simulink model "AHRS_voter_Harness1"  (R2018b)
settings: Solver=FixedStepDiscrete  StartTime=0.0  StopTime=10.0  FixedStep=0.01  RelTol=1e-3  EnableMultiTasking=on
Description:
  | Testing of a single valid AHRS.
settings Model: Creator=bpotter  LastModifiedBy=bpotter
settings DataIOCC: LimitDataPoints=on  SaveOutput=off  DSMLogging=off  InspectSignalLogs=on  SaveTime=off
settings OptimizationCC: BlockReduction=off  DefaultParameterBehavior=Inlined  InitFltsAndDblsToZero=on  EfficientFloat2IntCast=on  EfficientMapNaN2IntZero=off  LifeSpan=inf  MaxStackSize=inf
settings DebuggingCC: SignalInfNanChecking=error  SignalRangeChecking=error  ReadBeforeWriteMsg=EnableAllAsError  WriteAfterWriteMsg=EnableAllAsError  WriteAfterReadMsg=EnableAllAsError  AlgebraicLoopMsg=error  ArtificialAlgebraicLoopMsg=error  SaveWithDisabledLinksMsg=error  SaveWithParameterizedLinksMsg=error  BlockPriorityViolationMsg=error  SolverPrmCheckMsg=error  InheritedTsInSrcMsg=error  SigSpecEnsureSampleTimeMsg=error  CheckMatrixSingularityMsg=error  IntegerOverflowMsg=error  ParameterUnderflowMsg=error  ParameterPrecisionLossMsg=error  ParameterTunabilityLossMsg=error  UnderSpecifiedDataTypeMsg=error  UnnecessaryDatatypeConvMsg=warning  VectorMatrixConversionMsg=error  SignalLabelMismatchMsg=error  UnconnectedInputMsg=error  UnconnectedOutputMsg=error  UnconnectedLineMsg=error  SFcnCompatibilityMsg=error  BusObjectLabelMismatch=error  RootOutportRequireBusObject=error  AssertControl=DisableAll  AllowSymbolicDim=off  ModelReferenceIOMsg=error  ModelReferenceIOMismatchMessage=error  UnknownTsInhSupMsg=error  ModelReferenceDataLoggingMessage=error  StateNameClashWarn=warning  StrictBusMsg=ErrorOnBusTreatedAsVector  NonBusSignalsTreatedAsBus=error  SFInvalidInputDataAccessInChartInitDiag=error  SFTransitionOutsideNaturalParentDiag=error  SFUnreachableExecutionPathDiag=error  SFUndirectedBroadcastEventsDiag=error  SFTransitionActionBeforeConditionDiag=error  IntegerSaturationMsg=error
settings HardwareCC: ProdBitPerPointer=32  ProdBitPerSizeT=32  ProdBitPerPtrDiffT=32  ProdLargestAtomicFloat=None  ProdEndianess=Unspecified  ProdWordSize=32  ProdHWDeviceType=32-bit Generic  TargetIntDivRoundTo=Zero
settings ModelReferenceCC: PropagateSignalLabelsOutOfModel=off
settings SFSimCC: SimUseLocalCustomCode=off  MATLABDynamicMemAlloc=off
settings RTWCC: SystemTargetFile=ert.tlc  TemplateMakefile=ert_default_tmf  GenerateReport=on  RTWUseLocalCustomCode=off  IncludeHyperlinkInReport=on  LaunchReport=on  PortableWordSizes=on  GenerateTraceInfo=on  GenerateTraceReport=on  GenerateTraceReportSl=on  GenerateTraceReportSf=on  GenerateTraceReportEml=on
settings CodeAppCC: ForceParamTrailComments=on  IgnoreCustomStorageClasses=off  MangleLength=4  StateflowObjectComments=on  ReqsInCode=on
settings ERTTargetCC: UtilityFuncGeneration=Shared location  MultiwordLength=2048  GenerateSampleERTMain=on  IncludeMdlTerminateFcn=off  GeneratePreprocessorConditionals=Disable all  SuppressErrorStatus=on  SupportAbsoluteTime=off  SupportNonFinite=off  ParenthesesLevel=Maximum  GenerateSharedConstants=off  ERTCustomFileTemplate=example_file_process.tlc  PreserveExpressionOrder=on  PreserveIfCondition=on  ConvertIfToSwitch=off  SuppressUnreachableDefaultCases=off
settings ConfigComp: CovEnable=on  CovScope=ReferencedModels  CovIncludeTopModel=off  CovMetricSettings=dcmtrzoibe  CovHTMLOptions=-sRT=1 -sVT=0 -aTS=0 -bRG=1 -bTC=1 -hTR=1 -nFC=0 -nFD=1 -scm=1 -bcm=1 -xEv=0 -xEM=0  CovHtmlReporting=on  CovSaveCumulativeToWorkspaceVar=on  CovCumulativeVarName=AHRScovCumData  CovCumulativeReport=on  CovModelRefEnable=all  CovExternalEMLEnable=off  CovSFcnEnable=off  PSVerificationMode=BugFinder  PSResultDir=Bugfinder_results_$ModelName$  PSAutoStubLUT=off

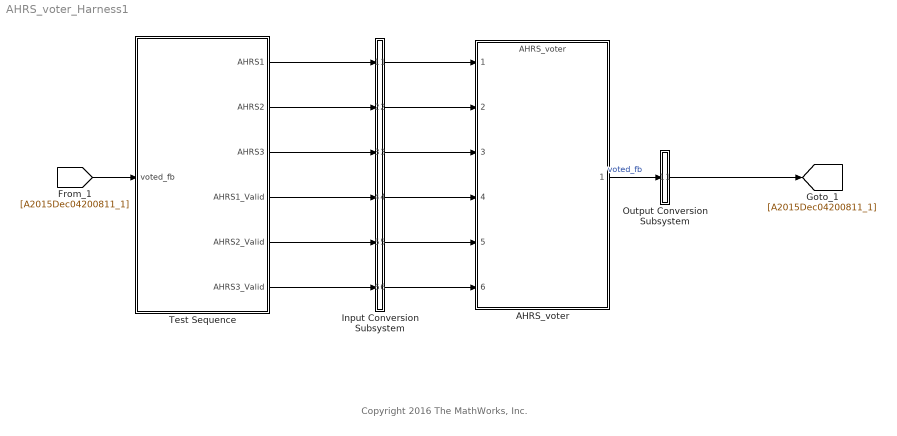
== system AHRS_voter_Harness1 ==
  note: Copyright 2016 The MathWorks, Inc.
  AHRS_voter : ModelReference  ModelNameDialog=AHRS_voter  SimulationMode=Normal  ModelReferenceVersion=1.56
  Input Conversion Subsystem : Subsystem  Tag=__SLT_ICS__
  Output Conversion Subsystem : Subsystem  Tag=__SLT_OCS__
  Test Sequence : Test Sequence  TreatAsAtomicUnit=on
  wires:
  [A2015Dec04200811_1] -> Test Sequence/1(voted_fb)
  Test Sequence/1(AHRS1) -> Input Conversion Subsystem/1(In_1)
  Test Sequence/2(AHRS2) -> Input Conversion Subsystem/2(In_2)
  Test Sequence/3(AHRS3) -> Input Conversion Subsystem/3(In_3)
  Test Sequence/4(AHRS1_Valid) -> Input Conversion Subsystem/4(In_4)
  Test Sequence/5(AHRS2_Valid) -> Input Conversion Subsystem/5(In_5)
  Test Sequence/6(AHRS3_Valid) -> Input Conversion Subsystem/6(In_6)
  Input Conversion Subsystem/1(Out_1) -> AHRS_voter/1
  Input Conversion Subsystem/2(Out_2) -> AHRS_voter/2
  Input Conversion Subsystem/3(Out_3) -> AHRS_voter/3
  Input Conversion Subsystem/4(Out_4) -> AHRS_voter/4
  Input Conversion Subsystem/5(Out_5) -> AHRS_voter/5
  Input Conversion Subsystem/6(Out_6) -> AHRS_voter/6
  AHRS_voter/1 -> Output Conversion Subsystem/1(In_1)  "voted_fb"
  Output Conversion Subsystem/1(Out_1) -> [A2015Dec04200811_1]

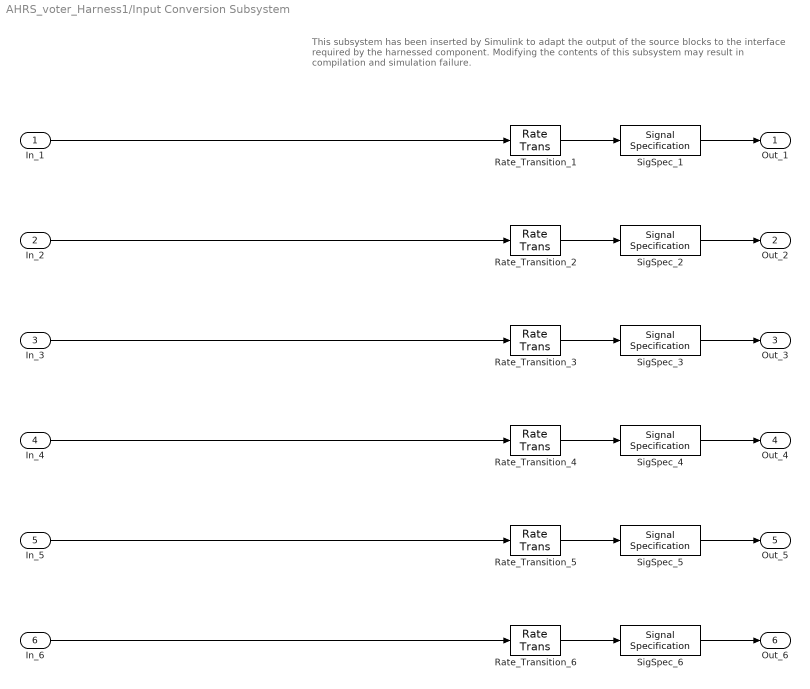
== system AHRS_voter_Harness1/Input Conversion Subsystem ==
  note: This subsystem has been inserted by Simulink to adapt the output of the source blocks to the interface required by the harnessed component.
      |  Modifying the contents of this subsystem may result in compilation and simulation failure.
  In_1 : Inport
  In_2 : Inport  Port=2
  In_3 : Inport  Port=3
  In_4 : Inport  Port=4
  In_5 : Inport  Port=5
  In_6 : Inport  Port=6
  Rate_Transition_{1..6} (6 alike) : RateTransition  OutPortSampleTime=0.01
  SigSpec_1 : SignalSpecification  OutDataTypeStr=double  Dimensions=[5]  SampleTime=0.01
  SigSpec_2 : SignalSpecification  OutDataTypeStr=double  Dimensions=[5]  SampleTime=0.01
  SigSpec_3 : SignalSpecification  OutDataTypeStr=double  Dimensions=[5]  SampleTime=0.01
  SigSpec_4 : SignalSpecification  OutDataTypeStr=boolean  Dimensions=[1]  SampleTime=0.01
  SigSpec_5 : SignalSpecification  OutDataTypeStr=boolean  Dimensions=[1]  SampleTime=0.01
  SigSpec_6 : SignalSpecification  OutDataTypeStr=boolean  Dimensions=[1]  SampleTime=0.01
  Out_1 : Outport
  Out_2 : Outport  Port=2
  Out_3 : Outport  Port=3
  Out_4 : Outport  Port=4
  Out_5 : Outport  Port=5
  Out_6 : Outport  Port=6
  wires:
  In_1/1 -> Rate_Transition_1/1
  In_2/1 -> Rate_Transition_2/1
  In_3/1 -> Rate_Transition_3/1
  In_4/1 -> Rate_Transition_4/1
  In_5/1 -> Rate_Transition_5/1
  In_6/1 -> Rate_Transition_6/1
  Rate_Transition_1/1 -> SigSpec_1/1
  Rate_Transition_2/1 -> SigSpec_2/1
  Rate_Transition_3/1 -> SigSpec_3/1
  Rate_Transition_4/1 -> SigSpec_4/1
  Rate_Transition_5/1 -> SigSpec_5/1
  Rate_Transition_6/1 -> SigSpec_6/1
  SigSpec_1/1 -> Out_1/1
  SigSpec_2/1 -> Out_2/1
  SigSpec_3/1 -> Out_3/1
  SigSpec_4/1 -> Out_4/1
  SigSpec_5/1 -> Out_5/1
  SigSpec_6/1 -> Out_6/1

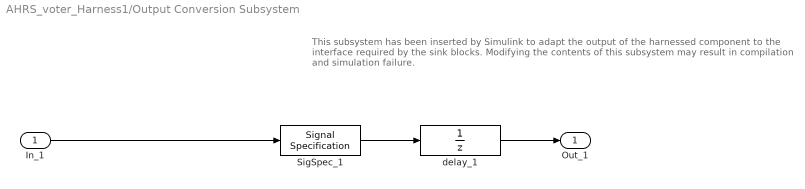
== system AHRS_voter_Harness1/Output Conversion Subsystem ==
  note: This subsystem has been inserted by Simulink to adapt the output of the harnessed component to the interface required by the sink blocks.
      |  Modifying the contents of this subsystem may result in compilation and simulation failure.
  In_1 : Inport
  SigSpec_1 : SignalSpecification  OutDataTypeStr=double  Dimensions=[5]  SampleTime=0.01
  delay_1 : UnitDelay  SampleTime=-1
  Out_1 : Outport
  wires:
  delay_1/1 -> Out_1/1
  SigSpec_1/1 -> delay_1/1
  In_1/1 -> SigSpec_1/1

== stateflow chart AHRS_voter_Harness1/Test Sequence ==
  settings: stateMachineType=SIMPLIFIED_MACHINE
  state step_1
    % Set each AHRS to have different data
    AHRS1 = ones(5, 1);
    AHRS2 = zeros(5, 1);
    AHRS3 = -ones(5, 1);
    % Set only AHRS1 to valid
    AHRS1_Valid = true;
    AHRS2_Valid = false;
    AHRS3_Valid = false;
  state step_2
    % Test that each element is using AHRS1 data
    verify(abs(voted_fb(1)-AHRS1(1))<Tol, ' AHRS1 Parameter1 selection failed');
    verify(abs(voted_fb(2)-AHRS1(2))<Tol, ' AHRS1 Parameter2 selection failed');
    verify(abs(voted_fb(3)-AHRS1(3))<Tol, ' AHRS1 Parameter3 selection failed');
    verify(abs(voted_fb(4)-AHRS1(4))<Tol, ' AHRS1 Parameter4 selection failed');
    verify(abs(voted_fb(5)-AHRS1(5))<Tol, ' AHRS1 Parameter5 selection failed');
  state step_3
    % Set only AHRS2 to valid
    AHRS1_Valid = false;
    AHRS2_Valid = true;
  state step_4
    % Test that each element is using AHRS2 data
    verify(abs(voted_fb(1)-AHRS2(1))<Tol, ' AHRS2 Parameter1 selection failed');
    verify(abs(voted_fb(2)-AHRS2(2))<Tol, ' AHRS2 Parameter2 selection failed');
    verify(abs(voted_fb(3)-AHRS2(3))<Tol, ' AHRS2 Parameter3 selection failed');
    verify(abs(voted_fb(4)-AHRS2(4))<Tol, ' AHRS2 Parameter4 selection failed');
    verify(abs(voted_fb(5)-AHRS2(5))<Tol, ' AHRS2 Parameter5 selection failed');
  state step_5
    % Set only AHRS3 to valid
    AHRS2_Valid = false;
    AHRS3_Valid = true;
  state step_6
    % Test that each element is using AHRS3 data
    verify(abs(voted_fb(1)-AHRS3(1))<Tol, ' AHRS3 Parameter1 selection failed');
    verify(abs(voted_fb(2)-AHRS3(2))<Tol, ' AHRS3 Parameter2 selection failed');
    verify(abs(voted_fb(3)-AHRS3(3))<Tol, ' AHRS3 Parameter3 selection failed');
    verify(abs(voted_fb(4)-AHRS3(4))<Tol, ' AHRS3 Parameter4 selection failed');
    verify(abs(voted_fb(5)-AHRS3(5))<Tol, ' AHRS3 Parameter5 selection failed');
  (default) -> step_1
  step_1 -> step_2 : [after(1, sec)]
  step_2 -> step_3
  step_3 -> step_4 : [after(1, sec)]
  step_4 -> step_5
  step_5 -> step_6 : [after(1, sec)]
  data: voted_fb input double size=[5]; AHRS1 output double size=[5]; AHRS2 output double size=[5]; AHRS3 output double size=[5]; AHRS1_Valid output boolean size=[1]; AHRS2_Valid output boolean size=[1]; AHRS3_Valid output boolean size=[1]; Tol constant double =1e-7
